simulink model "multifusion"  (R2023b)
settings: Solver=VariableStepAuto  StartTime=0.0  StopTime=10.0  RelTol=1e-3
undefined symbols (not defined in the file or in its folder): m, n
settings Model: Creator=anruk  LastModifiedBy=anruk

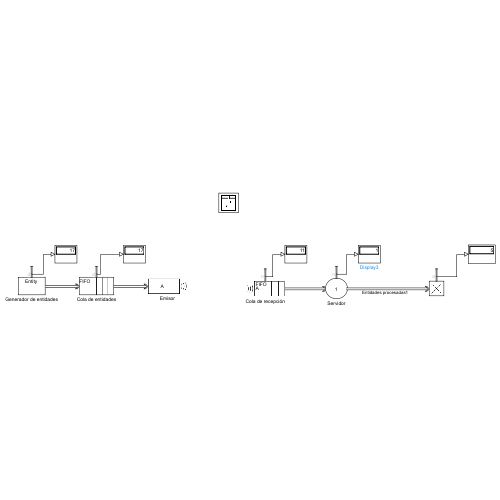
[thumbnail: Simulink's stored preview of the top-level diagram]
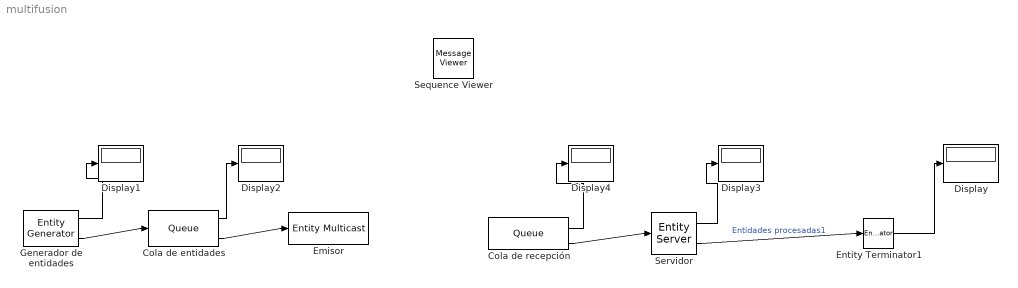
== system multifusion ==
  Cola de entidades : Queue  InputPortMessageModes=m  OutputPortMessageModes=n,m  NumberEntitiesDeparted=on
      settings: OutputPortMap=o0,o5
  Cola de recepción : Queue  OutputPortMessageModes=n,m  EntityArrivalSource=Multicast  NumberEntitiesInBlock=on
      settings: OutputPortMap=o1,o5
  Display{,1..4} (5 alike) : Display
  Emisor : EntityMulticast  Tag=A  InputPortMessageModes=m
  Entity Terminator1 : EntityTerminator  InputPortMessageModes=m  NumberEntitiesArrived=on
      settings: OutputPortMap=o0
  Generador de entidades : EntityGenerator  OutputPortMessageModes=n,m  TimeSource=MATLAB action  NumberEntitiesDeparted=on  EntityType=Structured  EntityTypeName=Entity
      settings: OutputPortMap=o0,o3
  Sequence Viewer : MessageViewer  History=1000  SavedRootId=#
  Servidor : EntityServer  InputPortMessageModes=m  OutputPortMessageModes=n,m  Capacity=1  ServiceTimeValue=2  NumberEntitiesInBlock=on
      settings: OutputPortMap=o1,o9
  wires:
  Cola de entidades/2 -> Emisor/1
  Generador de entidades/2 -> Cola de entidades/1
  Cola de recepción/2 -> Servidor/1
  Servidor/2 -> Entity Terminator1/1  "Entidades procesadas1"
  Entity Terminator1/1 -> Display/1
  Generador de entidades/1 -> Display1/1
  Cola de entidades/1 -> Display2/1
  Servidor/1 -> Display3/1
  Cola de recepción/1 -> Display4/1
